simulink model "P2"  (R2017a)
settings: Solver=ode45  StartTime=0.0  StopTime=10.0  RelTol=1e-3  EnableMultiTasking=on
settings Model: Creator=Gopanraj  LastModifiedBy=Soutrik
settings DataIOCC: LimitDataPoints=on  SaveFormat=Array  SignalLoggingSaveFormat=ModelDataLogs
settings OptimizationCC: ExpressionDepthLimit=2147483647  LifeSpan=inf
settings DebuggingCC: UnderspecifiedInitializationDetection=Classic  MergeDetectMultiDrivingBlocksExec=none  SolverPrmCheckMsg=warning  FcnCallInpInsideContextMsg=warning  StateNameClashWarn=warning  SFUnexpectedBacktrackingDiag=warning  SFNoUnconditionalDefaultTransitionDiag=warning  SFExecutionAtInitializationDiag=none
settings HardwareCC: ProdBitPerPointer=32  ProdBitPerSizeT=32  ProdBitPerPtrDiffT=32  ProdLargestAtomicFloat=None  ProdIntDivRoundTo=Undefined  ProdEndianess=Unspecified  ProdWordSize=32  ProdHWDeviceType=32-bit Generic
settings ModelReferenceCC: PropagateSignalLabelsOutOfModel=off
settings GRTTargetCC: TargetLangStandard=C89/C90 (ANSI)  GeneratePreprocessorConditionals=Disable all
settings ConfigComp: CovMetricSettings=dw  CovHtmlReporting=on  CovSaveCumulativeToWorkspaceVar=on  CovSaveSingleToWorkspaceVar=on  CovExternalEMLEnable=off

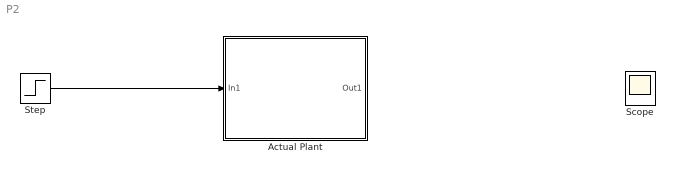
== system P2 ==
  Actual Plant : Subsystem
  Scope : Scope
  Step : Step  Time=0.1  After=5  SampleTime=0  VectorParams1D=off
  wires:
  Step/1 -> Actual Plant/1(In1)
  ? -> Scope/1

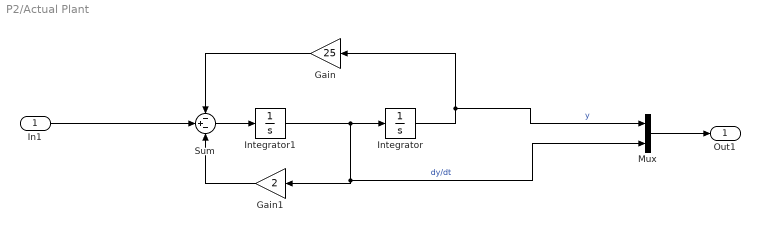
== system P2/Actual Plant ==
  In1 : Inport
  Gain : Gain  Gain=25
  Gain1 : Gain  Gain=2
  Integrator : Integrator
  Integrator1 : Integrator
  Mux : Mux  Inputs=2
  Sum : Sum  Inputs=-+-
  Out1 : Outport
  wires:
  Integrator1/1 -> Integrator/1, Mux/2, Gain1/1  "dy/dt"
  Gain1/1 -> Sum/3
  Sum/1 -> Integrator1/1
  In1/1 -> Sum/2
  Gain/1 -> Sum/1
  Integrator/1 -> Mux/1, Gain/1  "y"
  Mux/1 -> Out1/1
